simulink model "TrimIt"  (R2020a)
settings: Solver=VariableStepAuto  StartTime=0.0  StopTime=10.0  RelTol=1e-3
values from neighbouring files (symbols this model uses):
  psiP = 1    [init.m]
  zP = 0.1    [init.m]
settings Model: Creator=pelvoux1  LastModifiedBy=pelvoux1

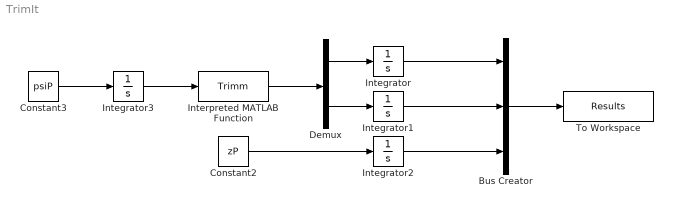
== system TrimIt ==
  Bus Creator : BusCreator  Inputs=3
  Constant2 : Constant  Value=zP
  Constant3 : Constant  Value=psiP
  Demux : Demux  Outputs=2
  Integrator{,1..3} (4 alike) : Integrator
  Interpreted MATLAB Function : MATLABFcn  MATLABFcn=Trimm  OutputDimensions=2  OutputSignalType=real
  To Workspace : ToWorkspace  VariableName=Results  SaveFormat=Timeseries  SampleTime=-1
  wires:
  Constant2/1 -> Integrator2/1
  Bus Creator/1 -> To Workspace/1
  Integrator/1 -> Bus Creator/1
  Integrator1/1 -> Bus Creator/2
  Integrator2/1 -> Bus Creator/3
  Constant3/1 -> Integrator3/1
  Integrator3/1 -> Interpreted MATLAB Function/1
  Demux/1 -> Integrator/1
  Demux/2 -> Integrator1/1
  Interpreted MATLAB Function/1 -> Demux/1
